simulink model "ex2_a"  (R2021a)
settings: Solver=VariableStepAuto  StartTime=0.0  StopTime=10.0  RelTol=1e-3

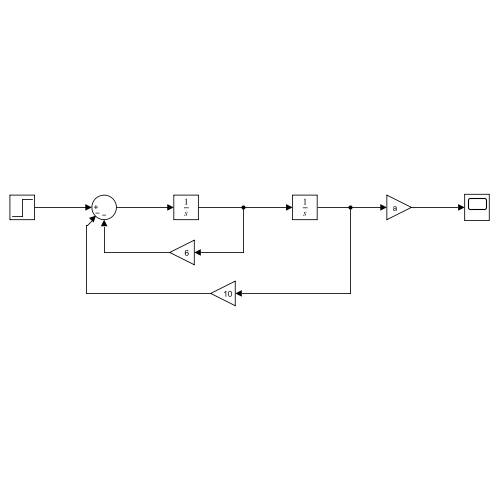
[thumbnail: Simulink's stored preview of the top-level diagram]
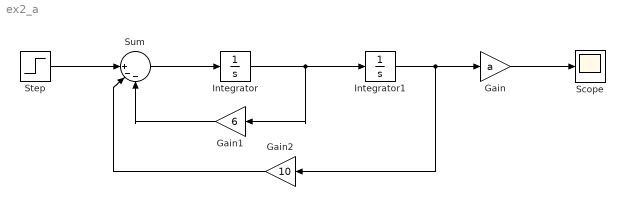
== system ex2_a ==
  Gain : Gain  Gain=a  mask{a=9}
      mask prompts: a "a="
  Gain1 : Gain  Gain=6
  Gain2 : Gain  Gain=10
  Integrator : Integrator
  Integrator1 : Integrator
  Scope : Scope
  Step : Step  SampleTime=0
  Sum : Sum  Inputs=||+--
  wires:
  Step/1 -> Sum/1
  Sum/1 -> Integrator/1
  Integrator/1 -> Gain1/1, Integrator1/1
  Integrator1/1 -> Gain2/1, Gain/1
  Gain/1 -> Scope/1
  Gain1/1 -> Sum/3
  Gain2/1 -> Sum/2
